simulink model "LQRsim_y_psi"  (R2021b)
settings: Solver=VariableStepAuto  StartTime=0.0  StopTime=10  RelTol=1e-3
settings Model: Creator=hty  LastModifiedBy=hty

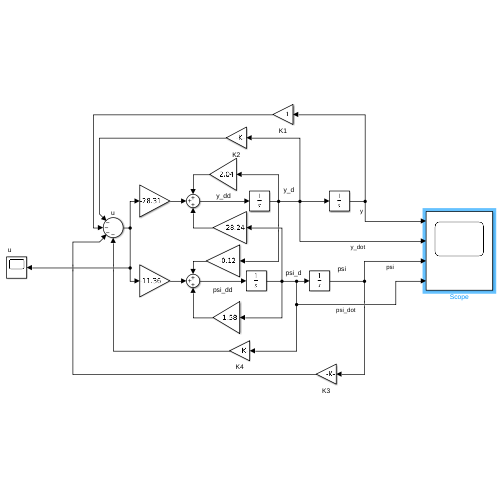
[thumbnail: Simulink's stored preview of the top-level diagram]
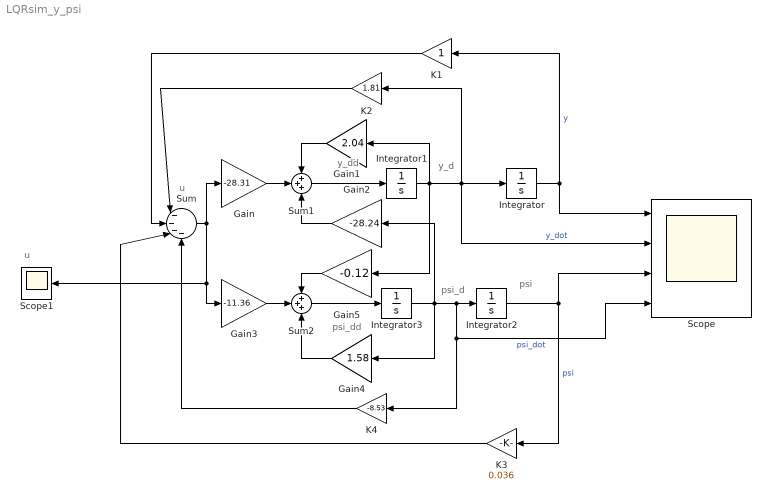
== system LQRsim_y_psi ==
  note: u
  note: y_d
  note: y_dd
  note: psi_d
  note: psi
  note: psi_dd
  note: u
  Gain : Gain  Gain=-28.31
  Gain1 : Gain  Gain=2.04
  Gain2 : Gain  Gain=-28.24
  Gain3 : Gain  Gain=-11.36
  Gain4 : Gain  Gain=1.58
  Gain5 : Gain  Gain=-0.12
  Integrator : Integrator  InitialCondition=5
  Integrator1 : Integrator
  Integrator2 : Integrator
  Integrator3 : Integrator
  K1 : Gain
  K2 : Gain  Gain=1.81
  K3 : Gain  Gain=0.036
  K4 : Gain  Gain=-8.53
  Scope : Scope  NumInputPorts=4
  Scope1 : Scope
  Sum : Sum  Inputs=|----
  Sum1 : Sum  Inputs=+++
  Sum2 : Sum  Inputs=+++
  wires:
  Integrator1/1 -> Gain5/1, Gain1/1, Scope/2, K2/1, Integrator/1  "y_dot"
  Integrator/1 -> K1/1, Scope/1  "y"
  Integrator3/1 -> Gain4/1, K4/1, Scope/4, Integrator2/1, Gain2/1  "psi_dot"
  Integrator2/1 -> K3/1, Scope/3  "psi"
  Sum2/1 -> Integrator3/1
  K2/1 -> Sum/1
  K1/1 -> Sum/2
  K4/1 -> Sum/4
  K3/1 -> Sum/3
  Sum/1 -> Gain3/1, Scope1/1, Gain/1
  Gain/1 -> Sum1/2
  Gain1/1 -> Sum1/1
  Gain2/1 -> Sum1/3
  Sum1/1 -> Integrator1/1
  Gain3/1 -> Sum2/2
  Gain4/1 -> Sum2/3
  Gain5/1 -> Sum2/1
